simulink model "giamsatpdmobongthanhslx"  (R2015a)
settings: Solver=ode45  SolverMode=SingleTasking  StartTime=0.0  StopTime=100  RelTol=1e-3
libraries: mblibv1 x12, fuzblock x1
settings Model: CovMetricSettings=dwe  CovHtmlReporting=off  covSaveCumulativeToWorkspaceVar=off  CovSaveSingleToWorkspaceVar=off  CovExternalEMLEnable=on  Creator=admin  LastModifiedBy=admin
settings DataIOCC: LimitDataPoints=off  SaveFormat=Dataset
settings DebuggingCC: SFUnexpectedBacktrackingDiag=error  SFNoUnconditionalDefaultTransitionDiag=error
settings HardwareCC: ProdBitPerPointer=64  ProdLargestAtomicFloat=Float  ProdIntDivRoundTo=Zero  ProdEndianess=LittleEndian  ProdHWDeviceType=Specified
settings ModelReferenceCC: PropagateSignalLabelsOutOfModel=on
settings SFSimCC: SimUseLocalCustomCode=on
settings RTWCC: RTWUseLocalCustomCode=on
settings GRTTargetCC: TargetLangStandard=C99 (ISO)  GeneratePreprocessorConditionals=Use local settings
settings SimMechanicsCC: VisDuringSimulation=on
settings ConfigurationSet: Description=Simscape Multibody

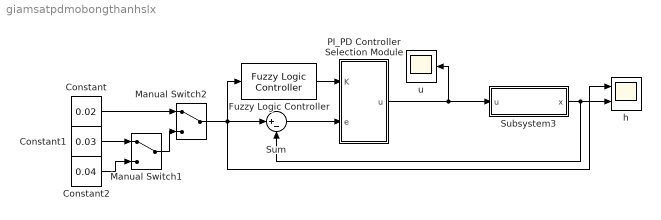
== system giamsatpdmobongthanhslx ==
  Constant : Constant  Value=0.02
  Constant1 : Constant  Value=0.03
  Constant2 : Constant  Value=0.04
  Fuzzy Logic Controller : fuzblock/Fuzzy Logic  Controller  FIS='fuzzypdobs.fis'
  Manual Switch1 : ManualSwitch
  Manual Switch2 : ManualSwitch
  PI_PD Controller Selection Module : Subsystem
  Subsystem3 : Subsystem
  Sum : Sum  Inputs=|+-
  h : Scope  NumInputPorts=2
      settings: TimeRange=auto  ShowLegends=on  MaxDataPoints=5000  YMin=-0.00494~-5  YMax=0.04442~5  SampleTime=-1
  u : Scope
      settings: TimeRange=auto  MaxDataPoints=5000  SaveToWorkspace=off  SaveName=ScopeData  YMin=-0.17153  YMax=0.15239  SampleTime=-1
  wires:
  Constant/1 -> Manual Switch2/1
  Sum/1 -> PI_PD Controller Selection Module/2(e)
  Constant1/1 -> Manual Switch1/1
  PI_PD Controller Selection Module/1(u) -> Subsystem3/1(u), u/1
  Manual Switch2/1 -> Fuzzy Logic Controller/1, h/1, Sum/1
  Subsystem3/1(x) -> h/2, Sum/2
  Fuzzy Logic Controller/1 -> PI_PD Controller Selection Module/1(K)
  Constant2/1 -> Manual Switch1/2
  Manual Switch1/1 -> Manual Switch2/2

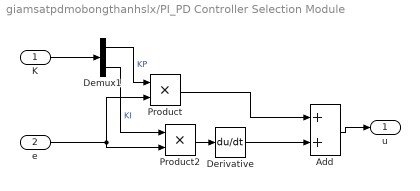
== system giamsatpdmobongthanhslx/PI_PD Controller Selection Module ==
  K : Inport
  e : Inport  Port=2
  Add : Sum
  Demux1 : Demux  Outputs=2
  Derivative : Derivative
  Product : Product
  Product2 : Product
  u : Outport
  wires:
  Add/1 -> u/1
  K/1 -> Demux1/1
  Demux1/1 -> Product/1  "KP"
  e/1 -> Product2/2, Product/2
  Product/1 -> Add/1
  Product2/1 -> Derivative/1
  Derivative/1 -> Add/2
  Demux1/2 -> Product2/1  "KI"

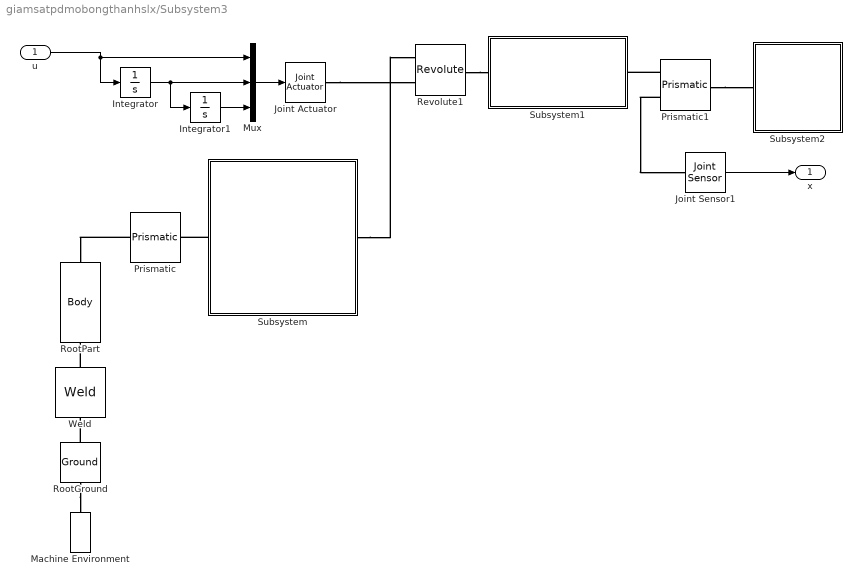
== system giamsatpdmobongthanhslx/Subsystem3 ==
  u : Inport
  Integrator : Integrator
  Integrator1 : Integrator
  Joint Actuator : mblibv1/Sensors &  Actuators/Joint Actuator  UpdateFromCAD=off  PhysicalDomain=Mechanical  PortType=blob  ActuationStyle=Motion  AngleUnits=rad  ArcVelocityUnits=rad/s  ArcAccelerationUnits=rad/s^2  CoordPositionUnits=m  VelocityUnits=m/s  AccelerationUnits=m/s^2  ForceUnits=N  TorqueUnits=N*m  ActiveIO=on  Width=3  DialogClass=MechanicalActuatorBlock  Primitive=R1  ReferenceFrame=Absolute (World)
  Joint Sensor1 : mblibv1/Sensors &  Actuators/Joint Sensor  UpdateFromCAD=off  PhysicalDomain=Mechanical  PortType=blob  Muxed=on  Pose=off  Angle=on  AngleUnits=deg  ArcVelocity=off  ArcVelocityUnits=deg/s  ArcAcceleration=off  ArcAccelerationUnits=deg/s^2  CoordPosition=on  CoordPositionUnits=m  Velocity=off  VelocityUnits=m/s  Acceleration=off  AccelerationUnits=m/s^2  Quaternion=on  QuaternionDT=off  QuaternionDDT=off  QuaternionUnits=off  OutputVector=[1]  ActiveIO=on  Width=1  DialogClass=MechanicalSensorBlock  Primitive=P1  Force=off  ForceUnits=N  Torque=off  TorqueUnits=N*m  ReferenceFrame=Absolute (World)  ReactionSensedSide=Follower  ReactionReferenceFrame=Absolute (World)  ReactionForce=off  ReactionForceUnits=N  ReactionMoment=off  ReactionMomentUnits=N*m
  Machine Environment : mblibv1/Bodies/Machine Environment  PortType=env  PhysicalDomain=Mechanical  DialogTemplateClass=MECH.MachineEnvironment  SyncWhenCopied=off  Gravity=[0 -9.81 0]  GravityUnits=m/s^2  GravityAsSignal=off  Dimensionality=Auto-detect  AnalysisType=Forward dynamics  LinearAssemblyTolerance=1e-3  LinearAssemblyToleranceUnits=m  AngularAssemblyTolerance=1e-3  AngularAssemblyToleranceUnits=rad  ConstraintSolverType=Stabilizing  ConstraintRelTolerance=1e-4  ConstraintAbsTolerance=1e-4  UseRobustSingularityHandling=off  RedundancyAnalysisToleranceType=Automatically select tolerance  RedundancyAnalysisTolerance=1e-14  StatePerturbationType=Fixed  PerturbationSize=1e-5  VisualizeMachine=on  BodyVisualizationType=Use model default body geometries  BodyColorSelMode=Use model default  DefaultBodyColor=[1 0 0]
  Mux : Mux  Inputs=3
  Prismatic : mblibv1/Joints/Prismatic  LConnTagsString=__newl0  RConnTagsString=__newr0  UpdateFromCAD=off  NumSAPorts=0  CutJoint=off  MarkAsCut=off  Primitives=prismatic  PrimitiveProps=P1$Base$[0 0 1]$prismatic  DialogClass=JointBlock  P1Axis=[0 0 1]
  Prismatic1 : mblibv1/Joints/Prismatic  LConnTagsString=__newl0|SA1  RConnTagsString=__newr0  UpdateFromCAD=off  NumSAPorts=1  CutJoint=off  MarkAsCut=off  Primitives=prismatic  PrimitiveProps=P1$Base$[1 0 0]$prismatic  DialogClass=JointBlock  P1Axis=[1 0 0]
  Revolute1 : mblibv1/Joints/Revolute  LConnTagsString=__newl0|SA1  RConnTagsString=__newr0  UpdateFromCAD=on  NumSAPorts=1  CutJoint=off  MarkAsCut=off  Primitives=prismatic  PrimitiveProps=R1$World$[0,0,-1]$revolute  DialogClass=JointBlock  R1Axis=[0,0,-1]
  RootGround : mblibv1/Bodies/Ground  UpdateFromCAD=on  LeftPortType=env  RightPortType=workingframe  PhysicalDomain=Mechanical  DialogClass=GroundBlock  CoordPosition=[7.39558e-007,-0.0451404,-0.0114254]  CoordPositionUnits=m  StateVectorMgrId=-1  MachineId=[0 0]  ShowEnvPort=on  ParameterChecksum=[1875868773, 3526601951, 134943748, 136016764]  TopologyChecksum=[630932490, 4066439718, 3395103115, 3545649823]
  RootPart : mblibv1/Bodies/Body  LConnTagsString=CS4  RConnTagsString=CS2  UpdateFromCAD=on  DialogClass=MechanicalBodyBlock  Mass=0  MassUnits=kg  InertiaUnits=kg*m^2  Inertia=[0,0,0;0,0,0;0,0,0]  Shape=Cylinder  ShapeDims=[1 1]  ShapeUnits=m  ShapeUse=false  Density=1  DensityUnits=kg/m^3  DensityUse=false  GraphicsMode=MACHINE_DEFAULT  BodyColorSelMode=MACHINE_DEFAULT  BodyColor=[1 0 0]  AttachedToCS=CS1  CG=Right$CG$[7.39558e-007 -0.0451404 -0.0114254]$WORLD$WORLD$m$[1 0 0;0 1 0;0 0 1]$3x3 Transform$rad$WORLD$false$none  WorkingFrames=Right$CS1$[0 0 0]$WORLD$WORLD$m$[1 0 0;0 1 0;0 0 1]$3x3 Transform$rad$WORLD$false$none#Right$CS2$[0 0 0]$WORLD$WORLD$m$[1 0 0;0 1 0;0 0 1]$3x3 Transform$rad$WORLD$true$none#Left$CS3$[0 0 0]$WORLD$WORLD$m$[1 0 0;0 1 0;0 0 1]$3x3 Transform$rad$WORLD$false$none#Left$CS4$[7.39558e-007 -0.0451404 -0.0114254]$WORLD$WORLD$m$[1 0 0;0 1 0;0 0 1]$3x3 Transform$rad$WORLD$true$none#Right$CS5$[7.39558e-007 -0.0451404 -0.0114254]$WORLD$WORLD$m$[1 0 0;0 1 0;0 0 1]$3x3 Transform$rad$WORLD$false$none  CGPos=[7.39558e-007 -0.0451404 -0.0114254]  CGRot=[1 0 0;0 1 0;0 0 1]  CS0Pos=[]  CS0Rot=[]  CS1Pos=[0 0 0]  CS1Rot=[1 0 0;0 1 0;0 0 1]  CS2Pos=[0 0 0]  CS2Rot=[1 0 0;0 1 0;0 0 1]  CS3Pos=[0 0 0]  CS3Rot=[1 0 0;0 1 0;0 0 1]  CS4Pos=[7.39558e-007 -0.0451404 -0.0114254]  CS4Rot=[1 0 0;0 1 0;0 0 1]  CS5Pos=[7.39558e-007 -0.0451404 -0.0114254]  CS5Rot=[1 0 0;0 1 0;0 0 1]  CS6Pos=[]  CS6Rot=[]  CS7Pos=[]  CS7Rot=[]  CS8Pos=[]  CS8Rot=[]  CS9Pos=[]  CS9Rot=[]  CS10Pos=[]  CS10Rot=[]  CS11Pos=[]  CS11Rot=[]  CS12Pos=[]  CS12Rot=[]  CS13Pos=[]  CS13Rot=[]  CS14Pos=[]  CS14Rot=[]  CS15Pos=[]  CS15Rot=[]  CS16Pos=[]  CS16Rot=[]  CS17Pos=[]  CS17Rot=[]  CS18Pos=[]  CS18Rot=[]  CS19Pos=[]  CS19Rot=[]  CS20Pos=[]  CS20Rot=[]
  Subsystem : Subsystem
      mask Display: image(imread('BaseMotor.jpg'))
  Subsystem1 : Subsystem
      mask Display: image(imread('Beam.jpg'))
  Subsystem2 : Subsystem
      mask Display: image(imread('Ball.jpg'))
  Weld : mblibv1/Joints/Weld  LConnTagsString=__newl0  RConnTagsString=__newr0  UpdateFromCAD=on  NumSAPorts=0  CutJoint=off  MarkAsCut=off  Primitives=weld  PrimitiveProps=W$World$[0.57735,0.57735,0.57735]$weld  DialogClass=JointBlock  WAxis=[0.57735,0.57735,0.57735]
  x : Outport
  wires:
  Integrator/1 -> Integrator1/1, Mux/2
  Integrator1/1 -> Mux/3
  Mux/1 -> Joint Actuator/1
  u/1 -> Integrator/1, Mux/1
  Joint Sensor1/1 -> x/1
  connections:
  Prismatic/LConn1 -- RootPart/RConn1
  Subsystem/LConn1 -- Prismatic/RConn1
  Prismatic1/RConn1 -- Subsystem2/LConn1
  RootGround/RConn1 -- Weld/LConn1
  Joint Actuator/RConn1 -- Revolute1/LConn2
  Revolute1/RConn1 -- Subsystem1/LConn1
  Prismatic1/LConn1 -- Subsystem1/RConn1
  Prismatic1/LConn2 -- Joint Sensor1/LConn1
  Subsystem/RConn1 -- Revolute1/LConn1
  Weld/RConn1 -- RootPart/LConn1
  RootGround/LConn1 -- Machine Environment/RConn1

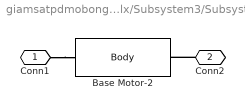
== system giamsatpdmobongthanhslx/Subsystem3/Subsystem ==
  Base Motor-2 : mblibv1/Bodies/Body  LConnTagsString=CS3  RConnTagsString=CS2  UpdateFromCAD=on  DialogClass=MechanicalBodyBlock  Mass=0.336571  MassUnits=kg  InertiaUnits=kg*m^2  Inertia=[0.000801363,3.96141e-010,3.99171e-015;3.96141e-010,0.000314607,0.000206003;3.99171e-015,0.000206003,0.000797116]  Shape=Cylinder  ShapeDims=[1 1]  ShapeUnits=m  ShapeUse=false  Density=1  DensityUnits=kg/m^3  DensityUse=false  GraphicsMode=GFXFILE  GraphicsFileName=BallBeam - Base Motor-1.STL  BodyColorSelMode=COLORPALETTE  BodyColor=[0.75294 0.75294 0.75294]  AttachedToCS=CS1  CG=Right$CG$[0 -0.0689193 -0.0170081]$WORLD$WORLD$m$[1 0 0;0 1 0;0 0 1]$3x3 Transform$rad$WORLD$false$none  WorkingFrames=Right$CS1$[0 0 -0.0592]$WORLD$WORLD$m$[1 0 0;0 1 0;0 0 1]$3x3 Transform$rad$WORLD$false$none#Right$CS2$[0 0 -0.00849566]$WORLD$WORLD$m$[1 0 0;0 1 0;0 0 1]$3x3 Transform$rad$WORLD$true$none#Left$CS3$[0 0 -0.0592]$WORLD$WORLD$m$[1 0 0;0 1 0;0 0 1]$3x3 Transform$rad$WORLD$true$none  CGPos=[0 -0.0689193 -0.0170081]  CGRot=[1 0 0;0 1 0;0 0 1]  CS0Pos=[]  CS0Rot=[]  CS1Pos=[0 0 -0.0592]  CS1Rot=[1 0 0;0 1 0;0 0 1]  CS2Pos=[0 0 -0.00849566]  CS2Rot=[1 0 0;0 1 0;0 0 1]  CS3Pos=[0 0 -0.0592]  CS3Rot=[1 0 0;0 1 0;0 0 1]  CS4Pos=[]  CS4Rot=[]  CS5Pos=[]  CS5Rot=[]  CS6Pos=[]  CS6Rot=[]  CS7Pos=[]  CS7Rot=[]  CS8Pos=[]  CS8Rot=[]  CS9Pos=[]  CS9Rot=[]  CS10Pos=[]  CS10Rot=[]  CS11Pos=[]  CS11Rot=[]  CS12Pos=[]  CS12Rot=[]  CS13Pos=[]  CS13Rot=[]  CS14Pos=[]  CS14Rot=[]  CS15Pos=[]  CS15Rot=[]  CS16Pos=[]  CS16Rot=[]  CS17Pos=[]  CS17Rot=[]  CS18Pos=[]  CS18Rot=[]  CS19Pos=[]  CS19Rot=[]  CS20Pos=[]  CS20Rot=[]
  Conn1 : PMIOPort  Side=Left
  Conn2 : PMIOPort  Port=2  Side=Right
  connections:
  Conn1/RConn1 -- Base Motor-2/LConn1
  Conn2/RConn1 -- Base Motor-2/RConn1

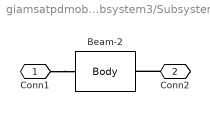
== system giamsatpdmobongthanhslx/Subsystem3/Subsystem1 ==
  Beam-2 : mblibv1/Bodies/Body  LConnTagsString=CS2  RConnTagsString=CS3  UpdateFromCAD=on  DialogClass=MechanicalBodyBlock  Mass=0.142403  MassUnits=kg  InertiaUnits=kg*m^2  Inertia=[1.38091e-005,0,-8.90739e-011;0,0.00336681,1.14658e-009;-8.90739e-011,1.14658e-009,0.00337387]  Shape=Cylinder  ShapeDims=[1 1]  ShapeUnits=m  ShapeUse=false  Density=1  DensityUnits=kg/m^3  DensityUse=false  GraphicsMode=GFXFILE  GraphicsFileName=BallBeam - Beam-2.STL  BodyColorSelMode=COLORPALETTE  BodyColor=[0.2 0.4 1]  AttachedToCS=CS1  CG=Right$CG$[2.60119e-006 0.000607844 1.32563e-005]$WORLD$WORLD$m$[0.999991 0.00427933 0;-0.00427933 0.999991 0;0 0 1]$3x3 Transform$rad$WORLD$false$none  WorkingFrames=Left$CS1$[0 0 0]$WORLD$WORLD$m$[0.999991 0.00427933 0;-0.00427933 0.999991 0;0 0 1]$3x3 Transform$rad$WORLD$false$none#Left$CS2$[0 0 -0.00849566]$World$World$m$[1 0 0;0 1 0;0 0 1]$3x3 Transform$rad$WORLD$true$none#Right$CS3$[0 0.0228707 0]$CG$WORLD$m$[1 0 0;0 1 0;0 0 1]$3x3 Transform$rad$WORLD$true$none  CGPos=[2.60119e-006 0.000607844 1.32563e-005]  CGRot=[0.999991 0.00427933 0;-0.00427933 0.999991 0;0 0 1]  CS0Pos=[]  CS0Rot=[]  CS1Pos=[0 0 0]  CS1Rot=[0.999991 0.00427933 0;-0.00427933 0.999991 0;0 0 1]  CS2Pos=[0 0 -0.00849566]  CS2Rot=[1 0 0;0 1 0;0 0 1]  CS3Pos=[0 0.0228707 0]  CS3Rot=[1 0 0;0 1 0;0 0 1]  CS4Pos=[]  CS4Rot=[]  CS5Pos=[]  CS5Rot=[]  CS6Pos=[]  CS6Rot=[]  CS7Pos=[]  CS7Rot=[]  CS8Pos=[]  CS8Rot=[]  CS9Pos=[]  CS9Rot=[]  CS10Pos=[]  CS10Rot=[]  CS11Pos=[]  CS11Rot=[]  CS12Pos=[]  CS12Rot=[]  CS13Pos=[]  CS13Rot=[]  CS14Pos=[]  CS14Rot=[]  CS15Pos=[]  CS15Rot=[]  CS16Pos=[]  CS16Rot=[]  CS17Pos=[]  CS17Rot=[]  CS18Pos=[]  CS18Rot=[]  CS19Pos=[]  CS19Rot=[]  CS20Pos=[]  CS20Rot=[]
  Conn1 : PMIOPort  Side=Left
  Conn2 : PMIOPort  Port=2  Side=Right
  connections:
  Conn1/RConn1 -- Beam-2/LConn1
  Conn2/RConn1 -- Beam-2/RConn1

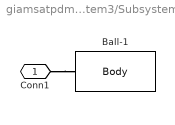
== system giamsatpdmobongthanhslx/Subsystem3/Subsystem2 ==
  Ball-1 : mblibv1/Bodies/Body  LConnTagsString=CS1  UpdateFromCAD=on  DialogClass=MechanicalBodyBlock  Mass=0.0218881  MassUnits=kg  InertiaUnits=kg*m^2  Inertia=[6.70322e-007,0,0;0,6.70322e-007,0;0,0,6.70322e-007]  Shape=Cylinder  ShapeDims=[1 1]  ShapeUnits=m  ShapeUse=false  Density=1  DensityUnits=kg/m^3  DensityUse=false  GraphicsMode=GFXFILE  GraphicsFileName=BallBeam - Ball-1.STL  BodyColorSelMode=COLORPALETTE  BodyColor=[0.8 0.8 0.8]  AttachedToCS=CG  CG=Right$CG$[0 0.0228707 0]$Adjoining$World$m$[1 0 0;0 -1 0;0 0 -1]$3x3 Transform$rad$WORLD$false$none  WorkingFrames=Left$CS2$[0 0.0228707 0]$Adjoining$World$m$[1 0 0;0 1 0;0 0 1]$3x3 Transform$rad$WORLD$false$none#Left$CS1$[0 0 0]$Adjoining$Adjoining$m$[1 0 0;0 1 0;0 0 1]$3x3 Transform$rad$WORLD$true$none  CGPos=[0 0.0228707 0]  CGRot=[1 0 0;0 -1 0;0 0 -1]  CS0Pos=[]  CS0Rot=[]  CS1Pos=[0 0 0]  CS1Rot=[1 0 0;0 1 0;0 0 1]  CS2Pos=[0 0.0228707 0]  CS2Rot=[1 0 0;0 1 0;0 0 1]  CS3Pos=[]  CS3Rot=[]  CS4Pos=[]  CS4Rot=[]  CS5Pos=[]  CS5Rot=[]  CS6Pos=[]  CS6Rot=[]  CS7Pos=[]  CS7Rot=[]  CS8Pos=[]  CS8Rot=[]  CS9Pos=[]  CS9Rot=[]  CS10Pos=[]  CS10Rot=[]  CS11Pos=[]  CS11Rot=[]  CS12Pos=[]  CS12Rot=[]  CS13Pos=[]  CS13Rot=[]  CS14Pos=[]  CS14Rot=[]  CS15Pos=[]  CS15Rot=[]  CS16Pos=[]  CS16Rot=[]  CS17Pos=[]  CS17Rot=[]  CS18Pos=[]  CS18Rot=[]  CS19Pos=[]  CS19Rot=[]  CS20Pos=[]  CS20Rot=[]
  Conn1 : PMIOPort  Side=Left
  connections:
  Conn1/RConn1 -- Ball-1/LConn1
